simulink model "Laboratorio3CasoB1"  (R2023a)
settings: Solver=VariableStepAuto  StartTime=0.0  StopTime=3/Frecuencia  RelTol=1e-3
undefined symbols (not defined in the file): Frecuencia, RR, VSPeakB
libraries: spsFourierLib x4, spsPowerLib x2, spsSeriesRLCBranchLib x2, spsMultimeterLib x1, spsLinearTransformerLib x1, spsACVoltageSourceLib x1, spspowerguiLib x1
settings Model: Creator=mluser  LastModifiedBy=Juan Esteban
settings OptimizationCC: ReuseModelBlockBuffer=off

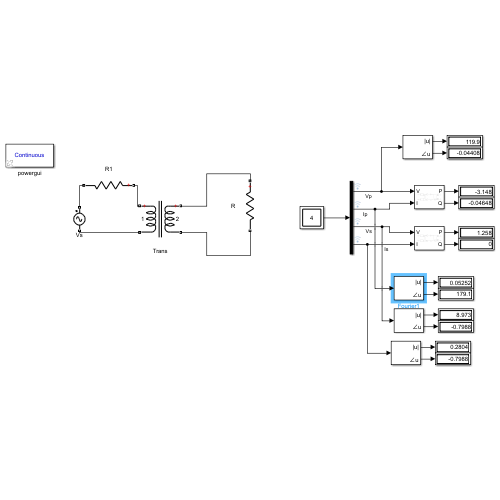
[thumbnail: Simulink's stored preview of the top-level diagram]
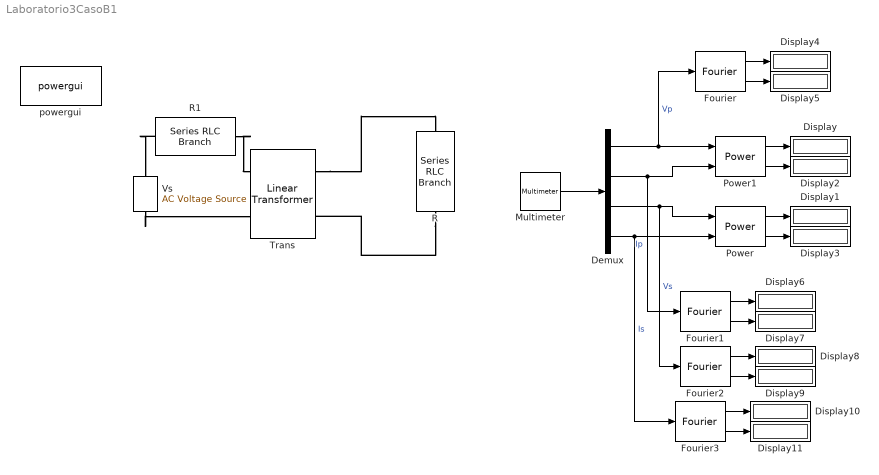
== system Laboratorio3CasoB1 ==
  Demux : Demux
  Display{,1..11} (12 alike) : Display
  Fourier{,1..3} (4 alike) : spsFourierLib/Fourier  Freq=60  n=1  InInit=[0, 0]  Ts=0
  Multimeter : spsMultimeterLib/Multimeter  L=11  sel=[3 6 1 5]  yselected={}  Gain=[1 1 1 1]  OutputType=Complex  PlotAtSimulationStop=off  PhasorSimulation=off
  Power : spsPowerLib/Power  Freq=60  Vinit=[1, 0]  Iinit=[1, 0]  Ts=0
  Power1 : spsPowerLib/Power  Freq=60  Vinit=[1, 0]  Iinit=[1, 0]  Ts=0
  R : spsSeriesRLCBranchLib/Series RLC Branch  LConnTagsString=__new0  RConnTagsString=__new0  BranchType=R  Resistance=RR  Inductance=1e-3  SetiL0=off  InitialCurrent=0  Capacitance=1e-6  Setx0=off  InitialVoltage=0  Measurements=Branch voltage and current
  R1 : spsSeriesRLCBranchLib/Series RLC Branch  LConnTagsString=__new0  RConnTagsString=__new0  BranchType=R  Resistance=1.8  Inductance=1e-3  SetiL0=off  InitialCurrent=0  Capacitance=1e-6  Setx0=off  InitialVoltage=0  Measurements=Branch voltage and current
  Trans : spsLinearTransformerLib/Linear Transformer  UNITS=SI  NominalPower=[ 250e6 60 ]  winding1="[120 5  0.08 ]"  winding2=[9 0 0]  ThreeWindings=off  winding3=[3.15e+05 0.7938 0.084225]  RmLm=[3800 3800]  Measurements=All voltages and currents  DataType=on
  Vs : spsACVoltageSourceLib/AC Voltage Source  Amplitude=VSPeakB  Phase=0  Frequency=Frecuencia  SampleTime=0  Measurements=None  BusType=swing  Pref=10e3  Qref=0  Qmin=-inf  Qmax=+inf
  powergui : spspowerguiLib/powergui  Priority=1  SimulationMode=Continuous  SampleTime=50e-6  frequency=60  Iterations=50  frequencyindice=60  Pbase=100e6  ErrMax=1e-4  UnitsV=kV  UnitsW=MW  buscounter=0  FunctionMessages=off  echomessages=off  EnableUseOfTLC=off  CurrentSourceSwitches=off  DisableSnubberDevices=off  DisableRonSwitches=off  DisableVfSwitches=off  DisplayEquations=off  AutomaticDiscreteSolvers=off  SolverType=Tustin/Backward Euler (TBE)  Interpol=off  ExternalGateDelay=off  methode=off  Ts=100  x0status=blocks  SPID=on  SwTol=0  HookPort=off  NonlinearTolerance=1e-4  nMaxIteration=100  ContinueOnMaxIteration=off  RestoreLinks=warning  ResistiveCurrentMeasurement=off  Frange=[0:2:500]  Ylog=off  Xlog=on  ShowGrid=off  save=off  variable=ZData  structure=0  ZoomFFT=off  StartTime=0.0  cycles=1  DisplayStyle=1  fundamental=60  FreqAxis=off  MaxFrequency=1000  frequencyindicesteady=1  RmsSteady=1  display=off
  wires:
  Multimeter/1 -> Demux/1
  Demux/3 -> Fourier2/1, Power/1  "Vs"
  Demux/4 -> Fourier3/1, Power/2  "Is"
  Demux/1 -> Fourier/1, Power1/1  "Vp"
  Demux/2 -> Fourier1/1, Power1/2  "Ip"
  Power1/1 -> Display/1
  Power1/2 -> Display2/1
  Power/2 -> Display3/1
  Power/1 -> Display1/1
  Fourier/2 -> Display5/1
  Fourier/1 -> Display4/1
  Fourier1/2 -> Display7/1
  Fourier1/1 -> Display6/1
  Fourier2/2 -> Display9/1
  Fourier2/1 -> Display8/1
  Fourier3/2 -> Display11/1
  Fourier3/1 -> Display10/1
  connections:
  Vs/LConn1 -- Trans/LConn2
  Trans/RConn1 -- R/LConn1
  R/RConn1 -- Trans/RConn2
  R1/LConn1 -- Trans/LConn1
  R1/RConn1 -- Vs/RConn1
